simulink model "RC4_CablesHaut"  (R2024b)
settings: Solver=VariableStepAuto  StartTime=0.0  StopTime=.4  RelTol=1e-3
values from neighbouring files (symbols this model uses):
  fv = 0    [parametres.m]
  Jm = 13.1/1000/10000    (= 1.31e-06)    [parametres.m]
  Kadapt = Kcapt/Rt    (= 52.1518917524)    [parametres.m]
  Kcapt = 8192/2/pi    (= 1303.79729381)    [parametres.m]
  Kcm = 25.5e-3    (= 0.0255)    [parametres.m]
  KCou_I = 900    [parametres.m]
  KCou_P = 2000    [parametres.m]
  KDSI = KPos_D*80/1000000    (= 0.0736)    [parametres.m]
  Kem = 1/(374 *2*pi/60)    (= 0.0255328785709)    [parametres.m]
  KPos_I = 270    [parametres.m]
  KPos_P = 215    [parametres.m]
  KPSI = KPos_P*10/1000    (= 2.15)    [parametres.m]
  Lm = 0.77e-3    (= 0.00077)    [parametres.m]
  r = 1/18    (= 0.0555555555556)    [parametres.m]
  Rm = 7.36    [parametres.m]
  Rt = 25    [parametres.m]
undefined symbols (not defined in the file or in its folder): les_bd_ts, les_bg_ts, les_hd_ts, les_hg_ts
settings Model: Creator=xpess  LastModifiedBy=xpess

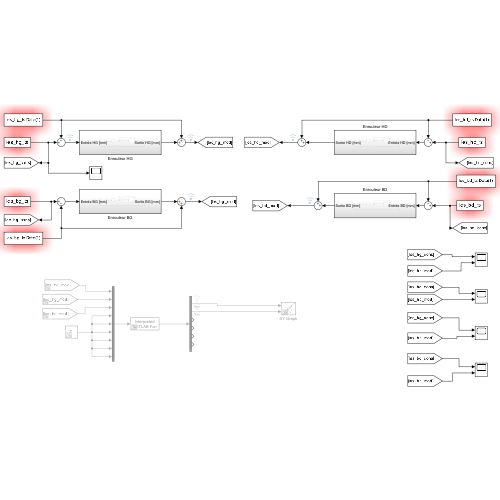
[thumbnail: Simulink's stored preview of the top-level diagram]
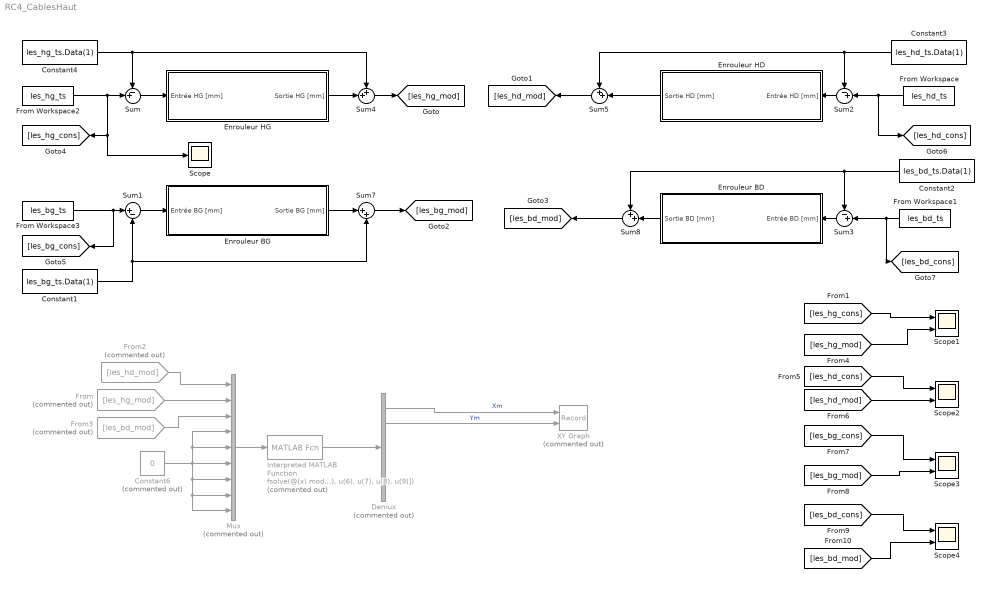
== system RC4_CablesHaut ==
  Constant1 : Constant  Value=les_bg_ts.Data(1)
  Constant2 : Constant  Value=les_bd_ts.Data(1)
  Constant3 : Constant  Value=les_hd_ts.Data(1)
  Constant4 : Constant  Value=les_hg_ts.Data(1)
  Constant6 : Constant  Commented=on  Value=0
  Demux : Demux  Commented=on  Outputs=6
  Enrouleur BD : Subsystem
  Enrouleur BG : Subsystem
  Enrouleur HD : Subsystem
  Enrouleur HG : Subsystem
  From : From  Commented=on  GotoTag=les_hg_mod
  From Workspace : FromWorkspace  VariableName=les_hd_ts
  From Workspace1 : FromWorkspace  VariableName=les_bd_ts
  From Workspace2 : FromWorkspace  VariableName=les_hg_ts
  From Workspace3 : FromWorkspace  VariableName=les_bg_ts
  From2 : From  Commented=on  GotoTag=les_hd_mod
  From3 : From  Commented=on  GotoTag=les_bd_mod
  Interpreted MATLAB Function : MATLABFcn  Commented=on  MATLABFcn=fsolve(@(x) modele_direct(x, [u(1),u(2),u(3)]), [u(4), u(5), u(6), u(7), u(8), u(9)])  OutputDimensions=6
  Mux : Mux  Commented=on  Inputs=9
  Scope : Scope
  Scope{1..4} (4 alike) : Scope  NumInputPorts=2
  Sum : Sum  Inputs=-+|
  Sum1 : Sum  Inputs=|+-
  Sum2 : Sum  Inputs=-+|
  Sum3 : Sum  Inputs=-+|
  Sum4 : Sum  Inputs=++|
  Sum5 : Sum  Inputs=++|
  Sum7 : Sum  Inputs=|++
  Sum8 : Sum  Inputs=++|
  XY Graph : Record  Commented=on  FileSettingsInternal="{\"entries\":[{\"content\":{\"excelSettings\":{\"content\":{},\"type\":\"Streamout.ExcelSettings\"}},\"type\":\"Streamout.FileSettingStorage\",\"uuid\":\"\"}],\"packageUris\":[\"http:\\/\\/schema.mathworks.com\\/mf0\\/streamout_blocks\\/R2020a\"],\"version\":\"1.0\"}"  Layout=[1 1]  SignalsInternal="{\"entries\":[{\"content\":{},\"type\":\"RecordBlkView.InputSignals\",\"uuid\":\"\"}],\"packageUris\":[\"http:\\/\\/schema.mathworks.com\\/mf0\\/streamout_blocks\\/R2020a\"],\"version\":\"1.0\"}"  VisualizationBindings="{\"xyplotplugin\":{\"info\":[{\"series\":[],\"subplotID\":1}]}}"  CompatibilityTag=XY
  wires:
  Sum/1 -> Enrouleur HG/1(Entrée HG [mm])
  From Workspace3/1 -> [les_bg_cons], Sum1/1
  Sum1/1 -> Enrouleur BG/1(Entrée BG [mm])
  From Workspace/1 -> Sum2/2, [les_hd_cons]
  Sum2/1 -> Enrouleur HD/1(Entrée HD [mm])
  Sum3/1 -> Enrouleur BD/1(Entrée BD [mm])
  From Workspace1/1 -> Sum3/2, [les_bd_cons]
  Constant2/1 -> Sum3/1, Sum8/1
  Constant4/1 -> Sum4/1, Sum/1
  Enrouleur HG/1(Sortie HG [mm]) -> Sum4/2
  Constant3/1 -> Sum2/1, Sum5/1
  Enrouleur HD/1(Sortie HD [mm]) -> Sum5/2
  Enrouleur BG/1(Sortie BG [mm]) -> Sum7/1
  Constant1/1 -> Sum7/2, Sum1/2
  Sum5/1 -> [les_hd_mod]
  Sum4/1 -> [les_hg_mod]
  Constant6/1 -> Mux/4, Mux/5, Mux/9, Mux/8, Mux/7, Mux/6
  Mux/1 -> Interpreted MATLAB Function/1
  Interpreted MATLAB Function/1 -> Demux/1
  Demux/1 -> XY Graph/1  "Xm"
  Demux/2 -> XY Graph/2  "Ym"
  Enrouleur BD/1(Sortie BD [mm]) -> Sum8/2
  From/1 -> Mux/2
  From2/1 -> Mux/1
  From3/1 -> Mux/3
  Sum7/1 -> [les_bg_mod]
  From Workspace2/1 -> [les_hg_cons], Scope/1, Sum/2
  Sum8/1 -> [les_bd_mod]
  [les_hg_cons] -> Scope1/1
  [les_hg_mod] -> Scope1/2
  [les_hd_cons] -> Scope2/1
  [les_hd_mod] -> Scope2/2
  [les_bg_cons] -> Scope3/1
  [les_bg_mod] -> Scope3/2
  [les_bd_cons] -> Scope4/1
  [les_bd_mod] -> Scope4/2

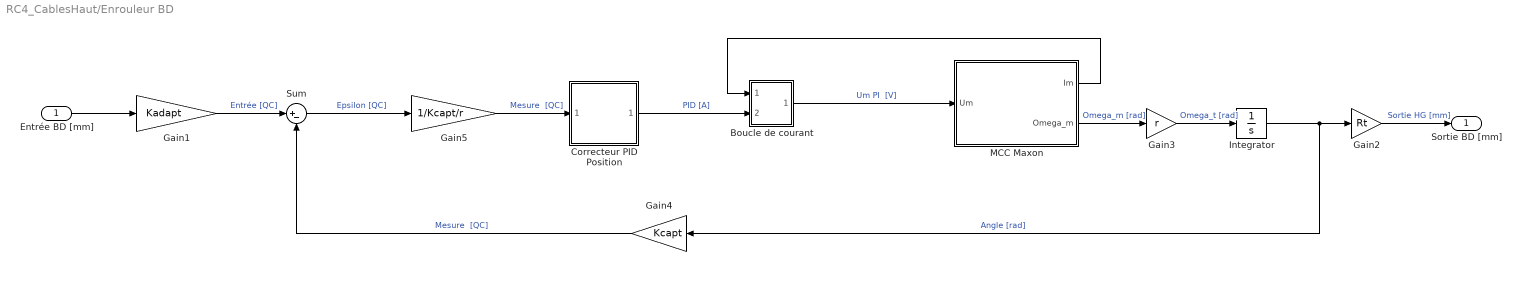
== system RC4_CablesHaut/Enrouleur BD ==
  Entrée BD [mm] : Inport
  Boucle de courant : Subsystem
      mask Display: image('EPOS.png');
  Correcteur PID Position : Subsystem
      mask Display: image('EPOS.png');
  Gain1 : Gain  Gain=Kadapt
  Gain2 : Gain  Gain=Rt
  Gain3 : Gain  Gain=r
  Gain4 : Gain  Gain=Kcapt
  Gain5 : Gain  Gain=1/Kcapt/r
  Integrator : Integrator
  MCC Maxon : Subsystem
      mask Display: image('MCC_1.png');
  Sum : Sum  Inputs=|+-
  Sortie BD [mm] : Outport
  wires:
  Sum/1 -> Gain5/1  "Epsilon [QC]"
  MCC Maxon/2(Omega_m) -> Gain3/1  "Omega_m [rad]"
  Gain3/1 -> Integrator/1  "Omega_t [rad]"
  Correcteur PID Position/1(Courant) -> Boucle de courant/2(Courant)  "PID [A]"
  Gain1/1 -> Sum/1  "Entrée [QC]"
  Boucle de courant/1(Out1) -> MCC Maxon/1(Um)  "Um PI  [V]"
  MCC Maxon/1(Im) -> Boucle de courant/1(In1)
  Gain5/1 -> Correcteur PID Position/1(Position)  "Mesure  [QC]"
  Integrator/1 -> Gain2/1, Gain4/1  "Angle [rad]"
  Gain4/1 -> Sum/2  "Mesure  [QC]"
  Entrée BD [mm]/1 -> Gain1/1
  Gain2/1 -> Sortie BD [mm]/1  "Sortie HG [mm]"

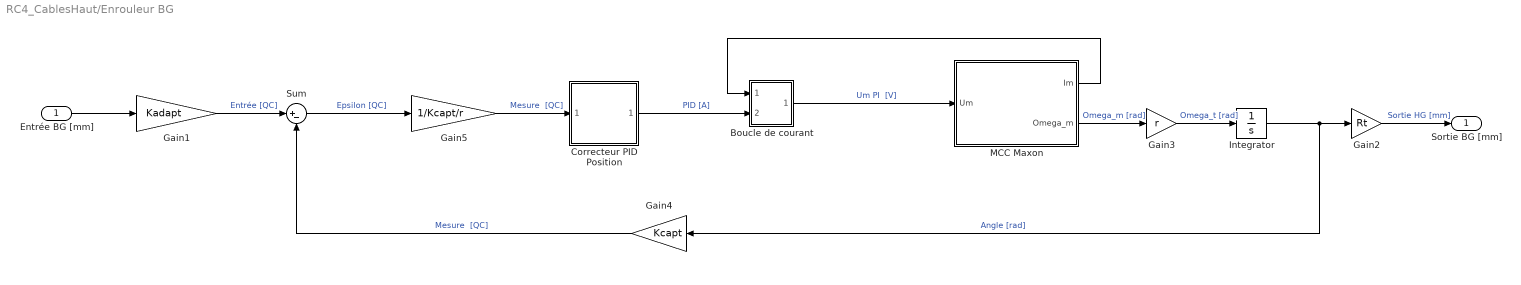
== system RC4_CablesHaut/Enrouleur BG ==
  Entrée BG [mm] : Inport
  Boucle de courant : Subsystem
      mask Display: image('EPOS.png');
  Correcteur PID Position : Subsystem
      mask Display: image('EPOS.png');
  Gain1 : Gain  Gain=Kadapt
  Gain2 : Gain  Gain=Rt
  Gain3 : Gain  Gain=r
  Gain4 : Gain  Gain=Kcapt
  Gain5 : Gain  Gain=1/Kcapt/r
  Integrator : Integrator
  MCC Maxon : Subsystem
      mask Display: image('MCC_1.png');
  Sum : Sum  Inputs=|+-
  Sortie BG [mm] : Outport
  wires:
  Gain2/1 -> Sortie BG [mm]/1  "Sortie HG [mm]"
  Entrée BG [mm]/1 -> Gain1/1
  Gain4/1 -> Sum/2  "Mesure  [QC]"
  Integrator/1 -> Gain4/1, Gain2/1  "Angle [rad]"
  Gain5/1 -> Correcteur PID Position/1(Position)  "Mesure  [QC]"
  MCC Maxon/1(Im) -> Boucle de courant/1(In1)
  Boucle de courant/1(Out1) -> MCC Maxon/1(Um)  "Um PI  [V]"
  Gain1/1 -> Sum/1  "Entrée [QC]"
  Correcteur PID Position/1(Courant) -> Boucle de courant/2(Courant)  "PID [A]"
  Gain3/1 -> Integrator/1  "Omega_t [rad]"
  MCC Maxon/2(Omega_m) -> Gain3/1  "Omega_m [rad]"
  Sum/1 -> Gain5/1  "Epsilon [QC]"

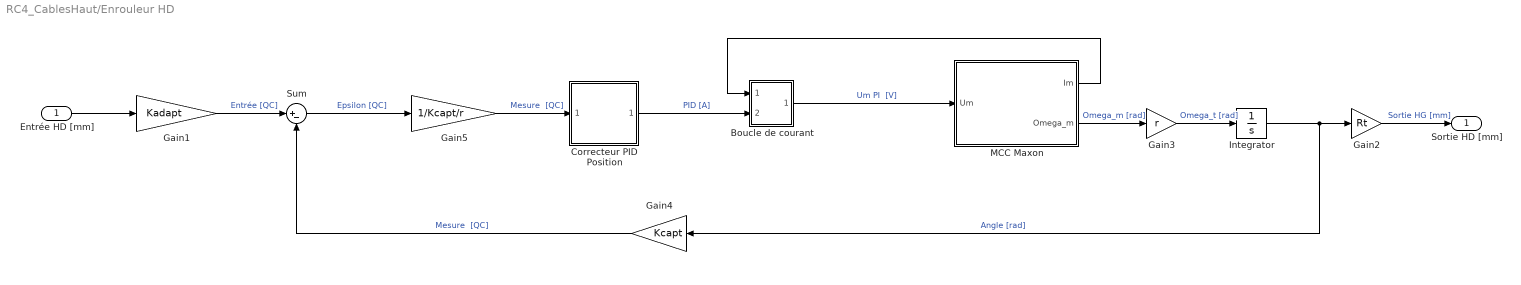
== system RC4_CablesHaut/Enrouleur HD ==
  Entrée HD [mm] : Inport
  Boucle de courant : Subsystem
      mask Display: image('EPOS.png');
  Correcteur PID Position : Subsystem
      mask Display: image('EPOS.png');
  Gain1 : Gain  Gain=Kadapt
  Gain2 : Gain  Gain=Rt
  Gain3 : Gain  Gain=r
  Gain4 : Gain  Gain=Kcapt
  Gain5 : Gain  Gain=1/Kcapt/r
  Integrator : Integrator
  MCC Maxon : Subsystem
      mask Display: image('MCC_1.png');
  Sum : Sum  Inputs=|+-
  Sortie HD [mm] : Outport
  wires:
  Gain2/1 -> Sortie HD [mm]/1  "Sortie HG [mm]"
  Entrée HD [mm]/1 -> Gain1/1
  Gain4/1 -> Sum/2  "Mesure  [QC]"
  Integrator/1 -> Gain4/1, Gain2/1  "Angle [rad]"
  Gain5/1 -> Correcteur PID Position/1(Position)  "Mesure  [QC]"
  MCC Maxon/1(Im) -> Boucle de courant/1(In1)
  Boucle de courant/1(Out1) -> MCC Maxon/1(Um)  "Um PI  [V]"
  Gain1/1 -> Sum/1  "Entrée [QC]"
  Correcteur PID Position/1(Courant) -> Boucle de courant/2(Courant)  "PID [A]"
  Gain3/1 -> Integrator/1  "Omega_t [rad]"
  MCC Maxon/2(Omega_m) -> Gain3/1  "Omega_m [rad]"
  Sum/1 -> Gain5/1  "Epsilon [QC]"

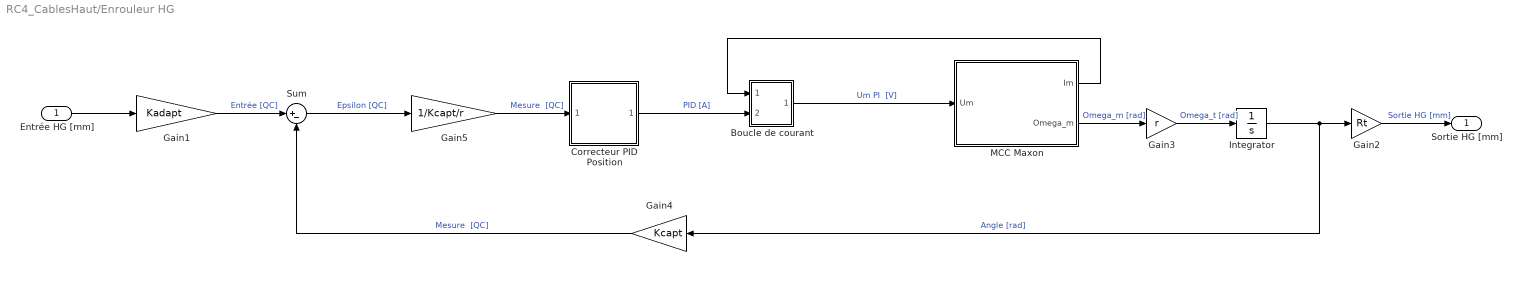
== system RC4_CablesHaut/Enrouleur HG ==
  Entrée HG [mm] : Inport
  Boucle de courant : Subsystem
      mask Display: image('EPOS.png');
  Correcteur PID Position : Subsystem
      mask Display: image('EPOS.png');
  Gain1 : Gain  Gain=Kadapt
  Gain2 : Gain  Gain=Rt
  Gain3 : Gain  Gain=r
  Gain4 : Gain  Gain=Kcapt
  Gain5 : Gain  Gain=1/Kcapt/r
  Integrator : Integrator
  MCC Maxon : Subsystem
      mask Display: image('MCC_1.png');
  Sum : Sum  Inputs=|+-
  Sortie HG [mm] : Outport
  wires:
  Sum/1 -> Gain5/1  "Epsilon [QC]"
  MCC Maxon/2(Omega_m) -> Gain3/1  "Omega_m [rad]"
  Gain3/1 -> Integrator/1  "Omega_t [rad]"
  Correcteur PID Position/1(Courant) -> Boucle de courant/2(Courant)  "PID [A]"
  Gain1/1 -> Sum/1  "Entrée [QC]"
  Boucle de courant/1(Out1) -> MCC Maxon/1(Um)  "Um PI  [V]"
  MCC Maxon/1(Im) -> Boucle de courant/1(In1)
  Gain5/1 -> Correcteur PID Position/1(Position)  "Mesure  [QC]"
  Integrator/1 -> Gain2/1, Gain4/1  "Angle [rad]"
  Gain4/1 -> Sum/2  "Mesure  [QC]"
  Entrée HG [mm]/1 -> Gain1/1
  Gain2/1 -> Sortie HG [mm]/1  "Sortie HG [mm]"

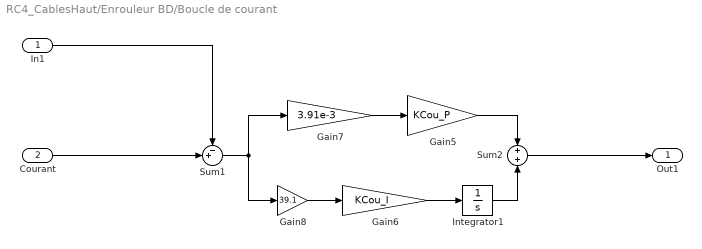
== system RC4_CablesHaut/Enrouleur BD/Boucle de courant ==
  In1 : Inport
  Courant : Inport  Port=2
  Gain5 : Gain  Gain=KCou_P
  Gain6 : Gain  Gain=KCou_I
  Gain7 : Gain  Gain=3.91e-3
  Gain8 : Gain  Gain=39.1
  Integrator1 : Integrator
  Sum1 : Sum  Inputs=-+|
  Sum2 : Sum  Inputs=+|+
  Out1 : Outport
  wires:
  Sum1/1 -> Gain7/1, Gain8/1
  Gain5/1 -> Sum2/1
  Sum2/1 -> Out1/1
  Integrator1/1 -> Sum2/2
  Gain8/1 -> Gain6/1
  In1/1 -> Sum1/1
  Gain7/1 -> Gain5/1
  Gain6/1 -> Integrator1/1
  Courant/1 -> Sum1/2

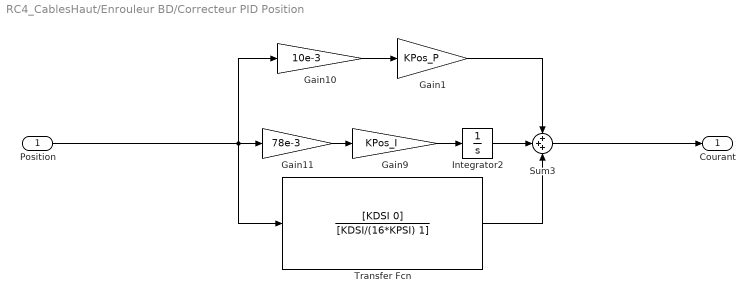
== system RC4_CablesHaut/Enrouleur BD/Correcteur PID Position ==
  Position : Inport
  Gain1 : Gain  Gain=KPos_P
  Gain10 : Gain  Gain=10e-3
  Gain11 : Gain  Gain=78e-3
  Gain9 : Gain  Gain=KPos_I
  Integrator2 : Integrator
  Sum3 : Sum  Inputs=+++
  Transfer Fcn : TransferFcn  Numerator=[KDSI 0]  Denominator=[KDSI/(16*KPSI) 1]
  Courant : Outport
  wires:
  Gain1/1 -> Sum3/1
  Position/1 -> Gain10/1, Transfer Fcn/1, Gain11/1
  Gain9/1 -> Integrator2/1
  Sum3/1 -> Courant/1
  Integrator2/1 -> Sum3/2
  Gain10/1 -> Gain1/1
  Gain11/1 -> Gain9/1
  Transfer Fcn/1 -> Sum3/3

== system RC4_CablesHaut/Enrouleur BD/MCC Maxon ==
  Um : Inport
  Gain : Gain  Gain=Kcm
  Gain1 : Gain  Gain=Kem
  Sum : Sum  Inputs=|+-
  Transfer Fcn : TransferFcn  Denominator=[Lm Rm]
  Transfer Fcn1 : TransferFcn  Denominator=[Jm fv]
  Im : Outport
  Omega_m : Outport  Port=2
  wires:
  Transfer Fcn/1 -> Im/1, Gain/1
  Transfer Fcn1/1 -> Omega_m/1, Gain1/1
  Gain/1 -> Transfer Fcn1/1
  Gain1/1 -> Sum/2
  Um/1 -> Sum/1
  Sum/1 -> Transfer Fcn/1

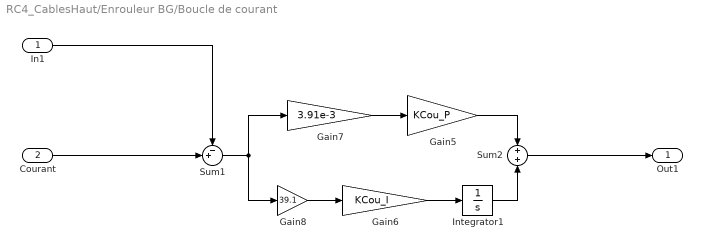
== system RC4_CablesHaut/Enrouleur BG/Boucle de courant ==
  In1 : Inport
  Courant : Inport  Port=2
  Gain5 : Gain  Gain=KCou_P
  Gain6 : Gain  Gain=KCou_I
  Gain7 : Gain  Gain=3.91e-3
  Gain8 : Gain  Gain=39.1
  Integrator1 : Integrator
  Sum1 : Sum  Inputs=-+|
  Sum2 : Sum  Inputs=+|+
  Out1 : Outport
  wires:
  Courant/1 -> Sum1/2
  Gain6/1 -> Integrator1/1
  Gain7/1 -> Gain5/1
  In1/1 -> Sum1/1
  Gain8/1 -> Gain6/1
  Integrator1/1 -> Sum2/2
  Sum2/1 -> Out1/1
  Gain5/1 -> Sum2/1
  Sum1/1 -> Gain8/1, Gain7/1

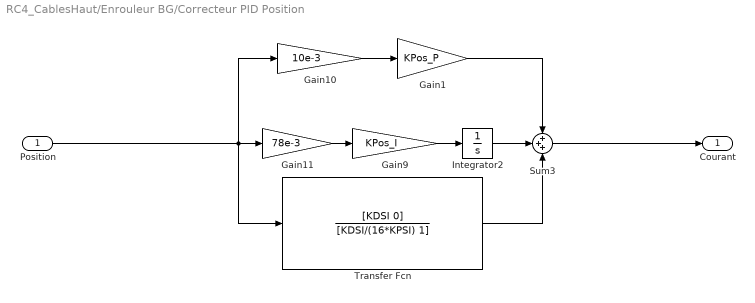
== system RC4_CablesHaut/Enrouleur BG/Correcteur PID Position ==
  Position : Inport
  Gain1 : Gain  Gain=KPos_P
  Gain10 : Gain  Gain=10e-3
  Gain11 : Gain  Gain=78e-3
  Gain9 : Gain  Gain=KPos_I
  Integrator2 : Integrator
  Sum3 : Sum  Inputs=+++
  Transfer Fcn : TransferFcn  Numerator=[KDSI 0]  Denominator=[KDSI/(16*KPSI) 1]
  Courant : Outport
  wires:
  Transfer Fcn/1 -> Sum3/3
  Gain11/1 -> Gain9/1
  Gain10/1 -> Gain1/1
  Integrator2/1 -> Sum3/2
  Sum3/1 -> Courant/1
  Gain9/1 -> Integrator2/1
  Position/1 -> Gain11/1, Transfer Fcn/1, Gain10/1
  Gain1/1 -> Sum3/1

== system RC4_CablesHaut/Enrouleur BG/MCC Maxon ==
  Um : Inport
  Gain : Gain  Gain=Kcm
  Gain1 : Gain  Gain=Kem
  Sum : Sum  Inputs=|+-
  Transfer Fcn : TransferFcn  Denominator=[Lm Rm]
  Transfer Fcn1 : TransferFcn  Denominator=[Jm fv]
  Im : Outport
  Omega_m : Outport  Port=2
  wires:
  Sum/1 -> Transfer Fcn/1
  Um/1 -> Sum/1
  Gain1/1 -> Sum/2
  Gain/1 -> Transfer Fcn1/1
  Transfer Fcn1/1 -> Gain1/1, Omega_m/1
  Transfer Fcn/1 -> Gain/1, Im/1

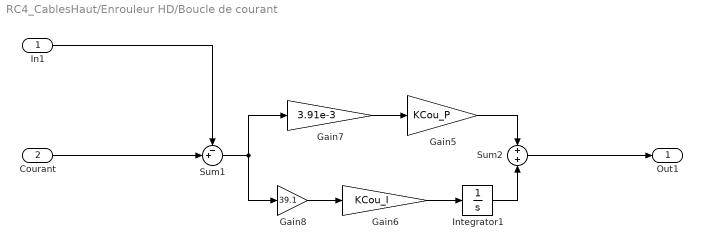
== system RC4_CablesHaut/Enrouleur HD/Boucle de courant ==
  In1 : Inport
  Courant : Inport  Port=2
  Gain5 : Gain  Gain=KCou_P
  Gain6 : Gain  Gain=KCou_I
  Gain7 : Gain  Gain=3.91e-3
  Gain8 : Gain  Gain=39.1
  Integrator1 : Integrator
  Sum1 : Sum  Inputs=-+|
  Sum2 : Sum  Inputs=+|+
  Out1 : Outport
  wires:
  Courant/1 -> Sum1/2
  Gain6/1 -> Integrator1/1
  Gain7/1 -> Gain5/1
  In1/1 -> Sum1/1
  Gain8/1 -> Gain6/1
  Integrator1/1 -> Sum2/2
  Sum2/1 -> Out1/1
  Gain5/1 -> Sum2/1
  Sum1/1 -> Gain8/1, Gain7/1

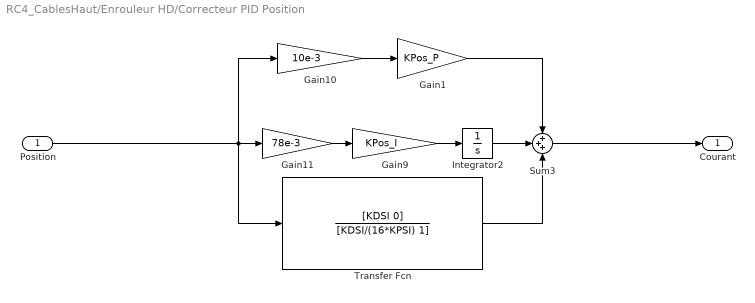
== system RC4_CablesHaut/Enrouleur HD/Correcteur PID Position ==
  Position : Inport
  Gain1 : Gain  Gain=KPos_P
  Gain10 : Gain  Gain=10e-3
  Gain11 : Gain  Gain=78e-3
  Gain9 : Gain  Gain=KPos_I
  Integrator2 : Integrator
  Sum3 : Sum  Inputs=+++
  Transfer Fcn : TransferFcn  Numerator=[KDSI 0]  Denominator=[KDSI/(16*KPSI) 1]
  Courant : Outport
  wires:
  Transfer Fcn/1 -> Sum3/3
  Gain11/1 -> Gain9/1
  Gain10/1 -> Gain1/1
  Integrator2/1 -> Sum3/2
  Sum3/1 -> Courant/1
  Gain9/1 -> Integrator2/1
  Position/1 -> Gain11/1, Transfer Fcn/1, Gain10/1
  Gain1/1 -> Sum3/1

== system RC4_CablesHaut/Enrouleur HD/MCC Maxon ==
  Um : Inport
  Gain : Gain  Gain=Kcm
  Gain1 : Gain  Gain=Kem
  Sum : Sum  Inputs=|+-
  Transfer Fcn : TransferFcn  Denominator=[Lm Rm]
  Transfer Fcn1 : TransferFcn  Denominator=[Jm fv]
  Im : Outport
  Omega_m : Outport  Port=2
  wires:
  Sum/1 -> Transfer Fcn/1
  Um/1 -> Sum/1
  Gain1/1 -> Sum/2
  Gain/1 -> Transfer Fcn1/1
  Transfer Fcn1/1 -> Gain1/1, Omega_m/1
  Transfer Fcn/1 -> Gain/1, Im/1

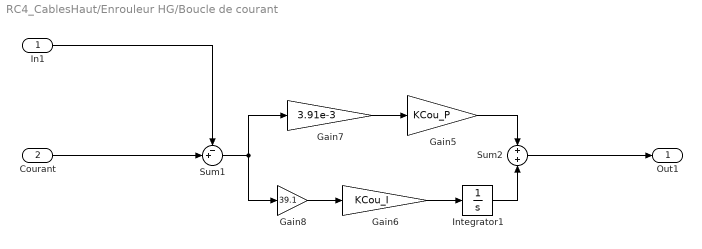
== system RC4_CablesHaut/Enrouleur HG/Boucle de courant ==
  In1 : Inport
  Courant : Inport  Port=2
  Gain5 : Gain  Gain=KCou_P
  Gain6 : Gain  Gain=KCou_I
  Gain7 : Gain  Gain=3.91e-3
  Gain8 : Gain  Gain=39.1
  Integrator1 : Integrator
  Sum1 : Sum  Inputs=-+|
  Sum2 : Sum  Inputs=+|+
  Out1 : Outport
  wires:
  Sum1/1 -> Gain7/1, Gain8/1
  Gain5/1 -> Sum2/1
  Sum2/1 -> Out1/1
  Integrator1/1 -> Sum2/2
  Gain8/1 -> Gain6/1
  In1/1 -> Sum1/1
  Gain7/1 -> Gain5/1
  Gain6/1 -> Integrator1/1
  Courant/1 -> Sum1/2

== system RC4_CablesHaut/Enrouleur HG/Correcteur PID Position ==
  Position : Inport
  Gain1 : Gain  Gain=KPos_P
  Gain10 : Gain  Gain=10e-3
  Gain11 : Gain  Gain=78e-3
  Gain9 : Gain  Gain=KPos_I
  Integrator2 : Integrator
  Sum3 : Sum  Inputs=+++
  Transfer Fcn : TransferFcn  Numerator=[KDSI 0]  Denominator=[KDSI/(16*KPSI) 1]
  Courant : Outport
  wires:
  Gain1/1 -> Sum3/1
  Position/1 -> Gain10/1, Transfer Fcn/1, Gain11/1
  Gain9/1 -> Integrator2/1
  Sum3/1 -> Courant/1
  Integrator2/1 -> Sum3/2
  Gain10/1 -> Gain1/1
  Gain11/1 -> Gain9/1
  Transfer Fcn/1 -> Sum3/3

== system RC4_CablesHaut/Enrouleur HG/MCC Maxon ==
  Um : Inport
  Gain : Gain  Gain=Kcm
  Gain1 : Gain  Gain=Kem
  Sum : Sum  Inputs=|+-
  Transfer Fcn : TransferFcn  Denominator=[Lm Rm]
  Transfer Fcn1 : TransferFcn  Denominator=[Jm fv]
  Im : Outport
  Omega_m : Outport  Port=2
  wires:
  Transfer Fcn/1 -> Im/1, Gain/1
  Transfer Fcn1/1 -> Omega_m/1, Gain1/1
  Gain/1 -> Transfer Fcn1/1
  Gain1/1 -> Sum/2
  Um/1 -> Sum/1
  Sum/1 -> Transfer Fcn/1
